simulink model "dcmotorss2"  (R2025b)
settings: Solver=VariableStepAuto  StartTime=0.0  StopTime=10.0  RelTol=1e-3
model workspace (MAT data in the model file):
  V_sup = Simulink.Parameter
  V_sup.Complexity = 'real'
  V_sup.Dimensions = [0 0]
  V_sup.DataType = 'auto'
  p = Simulink.Parameter
  p.Complexity = 'real'
  p.Dimensions = [0 0]
  p.DataType = 'auto'
  q = Simulink.Parameter
  q.Complexity = 'real'
  q.Dimensions = [0 0]
  q.DataType = 'auto'
  t = Simulink.Parameter
  t.Complexity = 'real'
  t.Dimensions = [0 0]
  t.DataType = 'auto'
  x = Simulink.Parameter
  x.Complexity = 'real'
  x.Dimensions = [0 0]
  x.DataType = 'auto'
  y = Simulink.Parameter
  y.Complexity = 'real'
  y.Dimensions = [0 0]
  y.DataType = 'auto'
  z = Simulink.Parameter
  z.Complexity = 'real'
  z.Dimensions = [0 0]
  z.DataType = 'auto'
undefined symbols (not defined in the file): b, J, K, L, R, T_ref, W_ref
libraries: pycoexlib x1
settings Model: Creator=adity

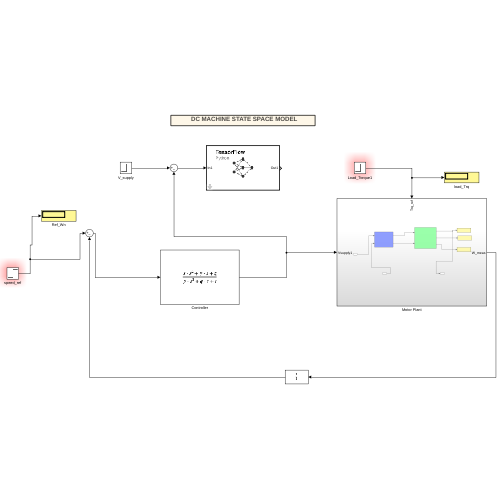
[thumbnail: Simulink's stored preview of the top-level diagram]
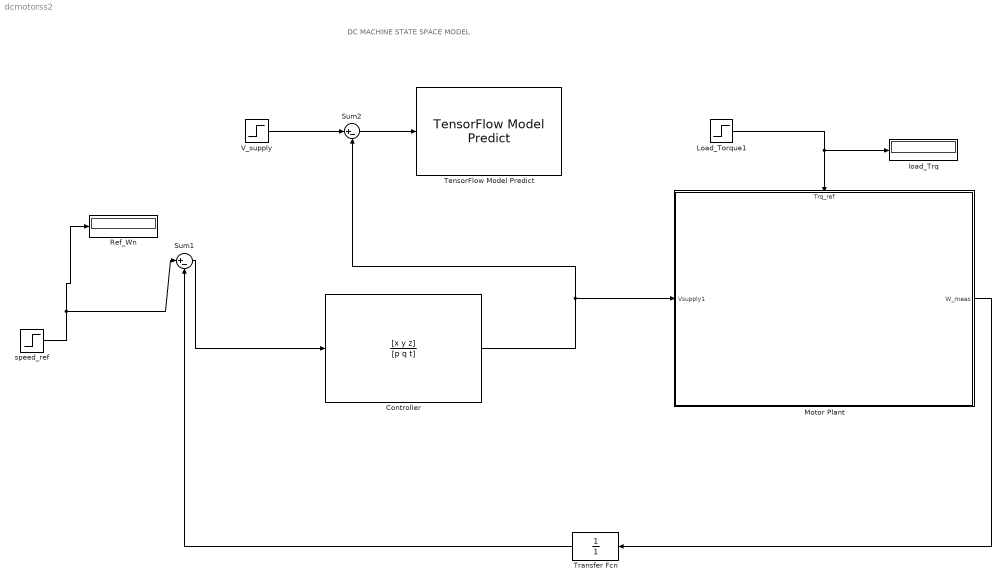
== system dcmotorss2 ==
  note: DC MACHINE STATE SPACE MODEL
  Controller : TransferFcn  Numerator=[x y z]  Denominator=[p q t]
  Load_Torque1 : Step  After=T_ref  SampleTime=0
  Motor Plant : Subsystem
      settings: PortSchema="{\"entries\":[{\"content\":{\"sides\":[{\"content\":{\"connectorIds\":[\"In1\"]},\"type\":\"ConnectorPlacement.EquallySpacedRectSide\",\"uuid\":\"e6cccd1e-7422-4dce-88f1-3af153357c6f\"},{\"content\":{\"connectorIds\":[\"Out1\"],\"side\":\"RIGHT\"},\"type\":\"ConnectorPlacement.EquallySpacedRectSide\",\"uuid\":\"0a9ab8b1-bfa0-4cb1-9483-d50c64dbd6ee\"},{\"content\":{\"connectorIds\":[\"In2\"],\"side\":\"TOP\"},\"type\":\"ConnectorPlacement.EquallySpacedRectSide\",\"uuid\":\"133b5cf7-1935-4674-a8a9-21a8bcdd933b\"}]},\"type\":\"ConnectorPlacement.EquallySpacedConnector\",\"uuid\":\"2e29a85c-43a3-45fc-a5d7-28468cf57ccf\"}],\"packageUris\":[\"http://schema.mathworks.com/mf0/Connector/R2020b\"],\"version\":\"1.0\"}"
  Ref_Wn : Display
  Sum1 : Sum  Inputs=|+-
  Sum2 : Sum  Inputs=|+-
  TensorFlow Model Predict : pycoexlib/TensorFlow Model Predict  ModelFile=untitled  InputTable={'In1','float32','',''}  OutputTable={'Out1','',''}  SampleTime=-1  InputDatatypes=float32  InputPermutations=[]  OutputPermutations=[]  PythonCoexecutionBlockType=TensorFlowModelBlock  VariableOutputMaxSizes=[]
  Transfer Fcn : TransferFcn  Denominator=[1]
  V_supply : Step  After=V_sup  SampleTime=0
  load_Trq : Display
  speed_ref : Step  After=W_ref  SampleTime=0
  wires:
  Load_Torque1/1 -> Motor Plant/2(Trq_ref), load_Trq/1
  speed_ref/1 -> Ref_Wn/1, Sum1/1
  Controller/1 -> Motor Plant/1(Vsupply1), Sum2/2
  Sum1/1 -> Controller/1
  Motor Plant/1(W_meas) -> Transfer Fcn/1
  Transfer Fcn/1 -> Sum1/2
  Sum2/1 -> TensorFlow Model Predict/1
  V_supply/1 -> Sum2/1

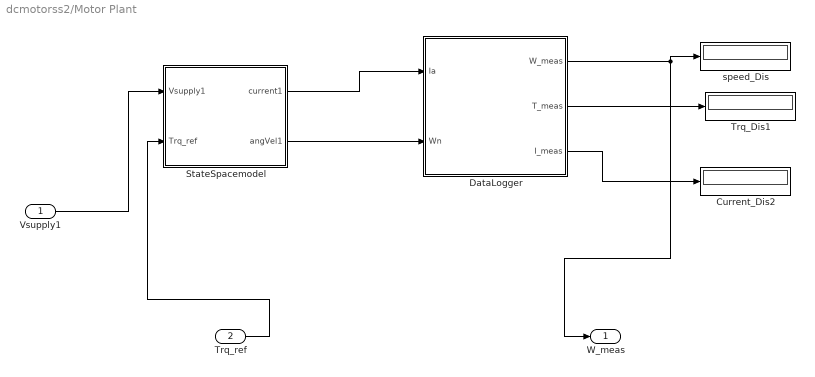
== system dcmotorss2/Motor Plant ==
  Vsupply1 : Inport
  Trq_ref : Inport  Port=2
  Current_Dis2 : Display
  DataLogger : Subsystem
  StateSpacemodel : Subsystem
  Trq_Dis1 : Display
  speed_Dis : Display
  W_meas : Outport
  wires:
  StateSpacemodel/1(current1) -> DataLogger/1(Ia)
  DataLogger/3(I_meas) -> Current_Dis2/1
  DataLogger/1(W_meas) -> W_meas/1, speed_Dis/1
  DataLogger/2(T_meas) -> Trq_Dis1/1
  StateSpacemodel/2(angVel1) -> DataLogger/2(Wn)
  Vsupply1/1 -> StateSpacemodel/1(Vsupply1)
  Trq_ref/1 -> StateSpacemodel/2(Trq_ref)

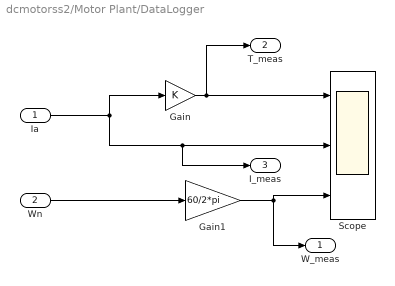
== system dcmotorss2/Motor Plant/DataLogger ==
  Ia : Inport
  Wn : Inport  Port=2
  Gain : Gain  Gain=K
  Gain1 : Gain  Gain=60/2*pi
  Scope : Scope  NumInputPorts=3
      settings: ActiveDisplayYMinimum=-1851.8596746326257  ActiveDisplayYMaximum=3301.7336749953711
  W_meas : Outport
  T_meas : Outport  Port=2
  I_meas : Outport  Port=3
  wires:
  Wn/1 -> Gain1/1
  Ia/1 -> Gain/1, I_meas/1, Scope/2
  Gain1/1 -> W_meas/1, Scope/3
  Gain/1 -> Scope/1, T_meas/1

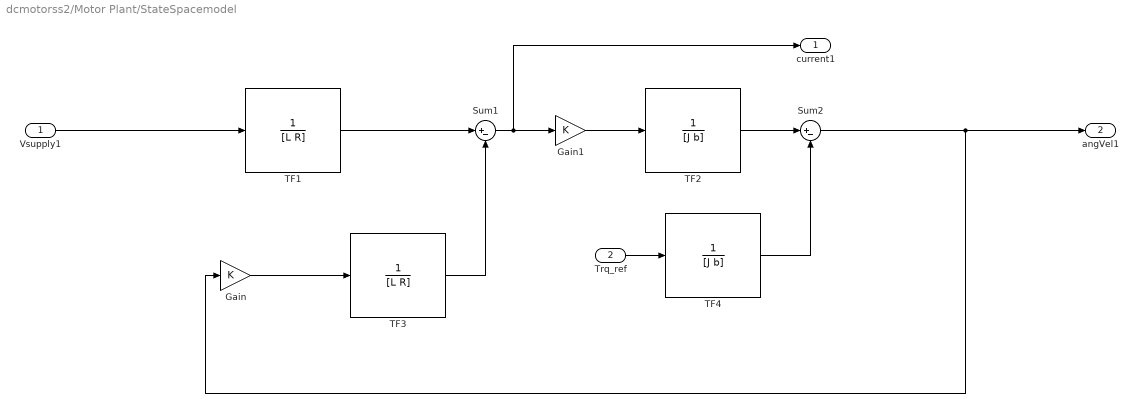
== system dcmotorss2/Motor Plant/StateSpacemodel ==
  Vsupply1 : Inport
  Trq_ref : Inport  Port=2
  Gain : Gain  Gain=K
  Gain1 : Gain  Gain=K
  Sum1 : Sum  Inputs=|+-
  Sum2 : Sum  Inputs=|+-
  TF1 : TransferFcn  Numerator=1  Denominator=[L R]
  TF2 : TransferFcn  Numerator=1  Denominator=[J b]
  TF3 : TransferFcn  Numerator=1  Denominator=[L R]
  TF4 : TransferFcn  Numerator=1  Denominator=[J b]
  current1 : Outport
  angVel1 : Outport  Port=2
  wires:
  Gain/1 -> TF3/1
  TF1/1 -> Sum1/1
  TF3/1 -> Sum1/2
  Sum1/1 -> Gain1/1, current1/1
  Gain1/1 -> TF2/1
  TF2/1 -> Sum2/1
  TF4/1 -> Sum2/2
  Sum2/1 -> angVel1/1, Gain/1
  Trq_ref/1 -> TF4/1
  Vsupply1/1 -> TF1/1
